simulink model "ctrl_lab"  (R2021b)
settings: Solver=VariableStepAuto  StartTime=0.0  StopTime=3  RelTol=1e-3
libraries: slrealtimeiplib x3, slrealtimeutilitieslib x2, slrealtimesharedmemorylib x2, slpidlib x1
settings Model: Creator=Jakob  LastModifiedBy=Jakob
settings DebuggingCC: UnconnectedInputMsg=none  UnconnectedOutputMsg=none  UnconnectedLineMsg=none
settings RTWCC: DLArmComputeVersion=20.02.1

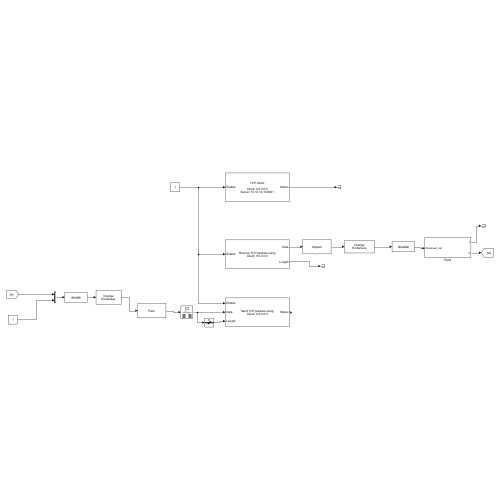
[thumbnail: Simulink's stored preview of the top-level diagram]
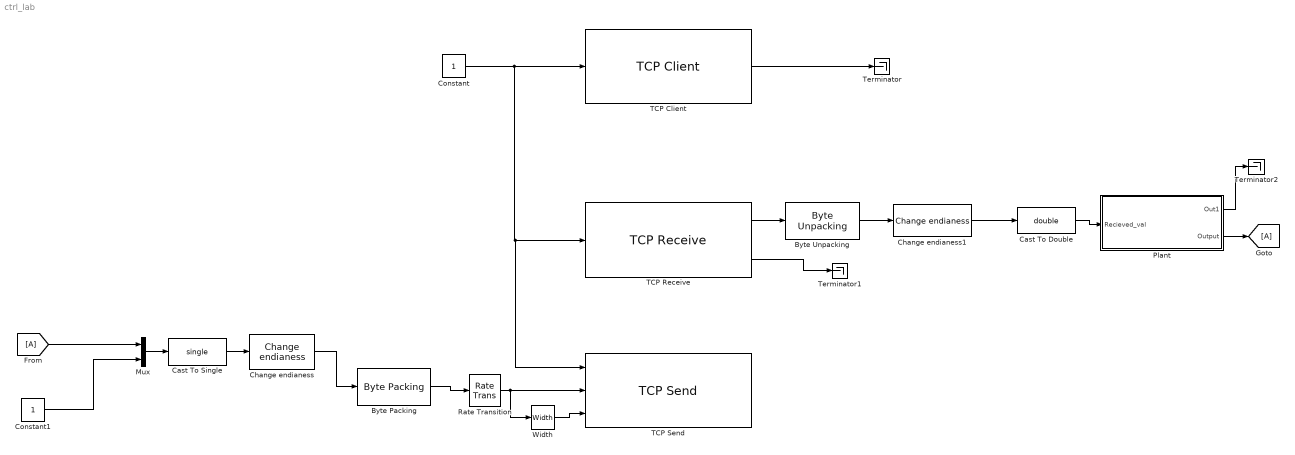
== system ctrl_lab ==
  Byte Packing : slrealtimeutilitieslib/Byte Packing  MaskPackedDataType=uint8  MaskUnpackedDataTypes={'single'}  MaskAlignment=1
  Byte Unpacking : slrealtimeutilitieslib/Byte Unpacking  MaskUnpackedDataTypes={'uint8'}  MaskUnpackedDataSizes={[2]}  MaskAlignment=1
      settings: SourceProductBaseCode=XP
  Cast To Double : DataTypeConversion  OutDataTypeStr=double
  Cast To Single : DataTypeConversion  OutDataTypeStr=single
  Change endianess : slrealtimesharedmemorylib/Change endianess  numInp=1  lengthIn=Byte
      settings: SourceProductBaseCode=XP
  Change endianess1 : slrealtimesharedmemorylib/Change endianess  numInp=1  lengthIn=Byte
      settings: SourceProductBaseCode=XP
  Constant : Constant
  Constant1 : Constant
  Mux : Mux  Inputs=2
  Plant : Subsystem
  Rate Transition : RateTransition  Deterministic=off  OutPortSampleTime=5e-3
  TCP Client : slrealtimeiplib/TCP Client  Priority=-1  useHostTargetConn=off  remoteAddress=10.10.10.10  remotePort=8001
      settings: SourceProductBaseCode=XP
  TCP Receive : slrealtimeiplib/TCP Receive  socketAddPortVal=Client: 0.0.0.0:0  rcvWidth=8  sampleTime=-1
      settings: SourceProductBaseCode=XP
  TCP Send : slrealtimeiplib/TCP Send  socketAddPortVal=Client: 0.0.0.0:0  sampleTime=-1
      settings: SourceProductBaseCode=XP
  Terminator : Terminator
  Terminator1 : Terminator
  Terminator2 : Terminator
  Width : Width
  wires:
  Constant/1 -> TCP Send/1, TCP Receive/1, TCP Client/1
  TCP Client/1 -> Terminator/1
  [A] -> Mux/1
  Constant1/1 -> Mux/2
  Mux/1 -> Cast To Single/1
  Cast To Single/1 -> Change endianess/1
  Change endianess/1 -> Byte Packing/1
  Byte Packing/1 -> Rate Transition/1
  Rate Transition/1 -> Width/1, TCP Send/2
  Width/1 -> TCP Send/3
  TCP Receive/1 -> Byte Unpacking/1
  Byte Unpacking/1 -> Change endianess1/1
  Change endianess1/1 -> Cast To Double/1
  TCP Receive/2 -> Terminator1/1
  Cast To Double/1 -> Plant/1(Recieved_val)
  Plant/2(Output) -> [A]
  Plant/1(Out1) -> Terminator2/1

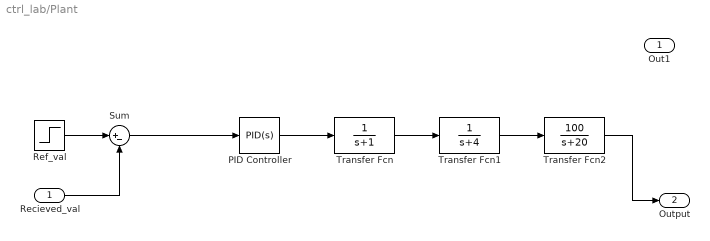
== system ctrl_lab/Plant ==
  Recieved_val : Inport
  PID Controller : slpidlib/PID Controller  Controller=PID  Form=Parallel  TimeDomain=Continuous-time  UseExternalTs=off  SampleTime=-1  IntegratorMethod=Forward Euler  FilterMethod=Forward Euler  ControllerParametersSource=internal  P=1  I=1  D=0  N=100  UseFilter=on  TunerSelectOption=Transfer Function Based (PID Tuner App)  InitialConditionSource=internal  InitialConditionForIntegrator=0  InitialConditionForFilter=0  DifferentiatorICPrevScaledInput=0  ExternalReset=none  TrackingMode=off  Kt=1  LimitOutput=off  SatLimitsSource=internal  UpperSaturationLimit=inf  LowerSaturationLimit=-inf  LinearizeAsGain=on  AntiWindupMode=none  Kb=1  POutMin=[]  POutMax=[]  IOutMin=[]  IOutMax=[]  DOutMin=[]  DOutMax=[]  NOutMin=[]  NOutMax=[]  SumOutMin=[]  SumOutMax=[]  SaturationOutMin=[]  SaturationOutMax=[]  PParamMin=[]  PParamMax=[]  IParamMin=[]  IParamMax=[]  DParamMin=[]  DParamMax=[]  NParamMin=[]  NParamMax=[]  KbParamMin=[]  KbParamMax=[]  KtParamMin=[]  KtParamMax=[]  KbOutMin=[]  KbOutMax=[]  KtOutMin=[]  KtOutMax=[]  IntegratorOutMin=[]  IntegratorOutMax=[]  FilterOutMin=[]  FilterOutMax=[]  SumI1OutMin=[]  SumI1OutMax=[]  SumI2OutMin=[]  SumI2OutMax=[]  SumI3OutMin=[]  SumI3OutMax=[]  SumI4OutMin=[]  SumI4OutMax=[]  SumDOutMin=[]  SumDOutMax=[]  DifferentiatorOutMin=[]  DifferentiatorOutMax=[]  FilterDiffOutCoefMin=[]  FilterDiffOutCoefMax=[]  ReciprocalOutMin=[]  ReciprocalOutMax=[]  SumDenOutMin=[]  SumDenOutMax=[]  SumNumOutMin=[]  SumNumOutMax=[]  DivideOutMin=[]  DivideOutMax=[]  UdiffTsProdOutMin=[]  UdiffTsProdOutMax=[]  NTsProdOutMin=[]  NTsProdOutMax=[]  UintegralTsProdOutMin=[]  UintegralTsProdOutMax=[]  UngainTsProdOutMin=[]  UngainTsProdOutMax=[]  IntegratorContinuousStateAttributes=''  IntegratorStateMustResolveToSignalObject=off  IntegratorRTWStateStorageClass=Auto  FilterContinuousStateAttributes=''  FilterStateMustResolveToSignalObject=off  FilterRTWStateStorageClass=Auto  ParallelPVariant=InternalParameters  IdealPVariant=Disabled  IVariant=InternalParameters  DVariant=InternalParameters  IntegratorVariant=Continuous  SatVariant=Disabled  AWVariant=Passthrough  PCopyVariant=Disabled  TRVariant=Disabled  FdbkBlocksVariant=Forward  IdealPFdbkVariant=Disabled  SatFdbkVariant=Disabled  DerivativeFilterVariant=ContFilter  NVariant=InternalParameters  NCopyVariant=Disabled  FilterICVariant=InternalICsFilter  IntegratorICVariant=InternalICs  ExternalResetVariant=Disabled  TRSumVariant=Passthrough  SumFdbkVariant=Disabled  SumVariant=Sum_PID  TsampFilterVariant=InternalTs  TsampNgainVariant=Passthrough  TsampIntegralVariant=Passthrough  ExternalSaturationOutDataTypeStr=Inherit: Same as second input
  Ref_val : Step  SampleTime=0
  Sum : Sum  Inputs=|+-
  Transfer Fcn : TransferFcn  Denominator=[1 1]
  Transfer Fcn1 : TransferFcn  Denominator=[1 4]
  Transfer Fcn2 : TransferFcn  Numerator=[100]  Denominator=[1 20]
  Out1 : Outport
  Output : Outport  Port=2
  wires:
  Ref_val/1 -> Sum/1
  Recieved_val/1 -> Sum/2
  Sum/1 -> PID Controller/1
  PID Controller/1 -> Transfer Fcn/1
  Transfer Fcn/1 -> Transfer Fcn1/1
  Transfer Fcn1/1 -> Transfer Fcn2/1
  Transfer Fcn2/1 -> Output/1
